simulink model "MPPT_RotEnc_Model1"  (R2018b)
settings: Solver=VariableStepAuto  StartTime=0.0  StopTime=1  RelTol=1e-3  AbsTol=1e-3  EnableMultiTasking=on
values from neighbouring files (symbols this model uses):
  ADC = 1024/5    (= 204.8)    [MPPT_RotEnc_Model.m]
  Cb = 400e-6    (= 0.0004)    [MPPT_RotEnc_Model.m]
  f = 10000    [MPPT_RotEnc_Model.m]
  lambda_pm = 1    [MPPT_RotEnc_Model.m]
  Lb = 1e-3    (= 0.001)    [MPPT_RotEnc_Model.m]
  Ls = 1    [MPPT_RotEnc_Model.m]
  p = 1    [MPPT_RotEnc_Model.m]
  R1 = 200e3    (= 200000)    [MPPT_RotEnc_Model.m]
  R2 = 100e3    (= 100000)    [MPPT_RotEnc_Model.m]
  Rl = 100    [MPPT_RotEnc_Model.m]
  Rs = 1    [MPPT_RotEnc_Model.m]
  Te = 1    [MPPT_RotEnc_Model.m]
  Wc = 1    [MPPT_RotEnc_Model.m]
libraries: powerlib x16, fl_lib x9, nesl_utility x5, elec_lib x1, pe_lib x1
settings Model: Creator=Cyrus  LastModifiedBy=Cyrus
settings SolverCC: AutoScaleAbsTol=off
settings DataIOCC: LimitDataPoints=on  MaxDataPoints=10000
settings OptimizationCC: LifeSpan=inf
settings DebuggingCC: AllowSymbolicDim=off  LibraryContextMissingDiagnostic=none  SFUnexpectedBacktrackingDiag=warning  SFNoUnconditionalDefaultTransitionDiag=warning  SFExecutionAtInitializationDiag=none
settings SFSimCC: SimUseLocalCustomCode=off
settings RTWCC: RTWUseLocalCustomCode=off
settings CodeAppCC: StateflowObjectComments=on
settings GRTTargetCC: TargetLangStandard=C89/C90 (ANSI)  GeneratePreprocessorConditionals=Disable all
settings ConfigComp: CovMetricSettings=dw  CovHtmlReporting=on  CovSaveCumulativeToWorkspaceVar=on  CovSaveSingleToWorkspaceVar=on  CovExternalEMLEnable=off  CovSFcnEnable=off
settings SimscapeCC: SimscapeLogType=all  SimscapeLogDataHistory=10000

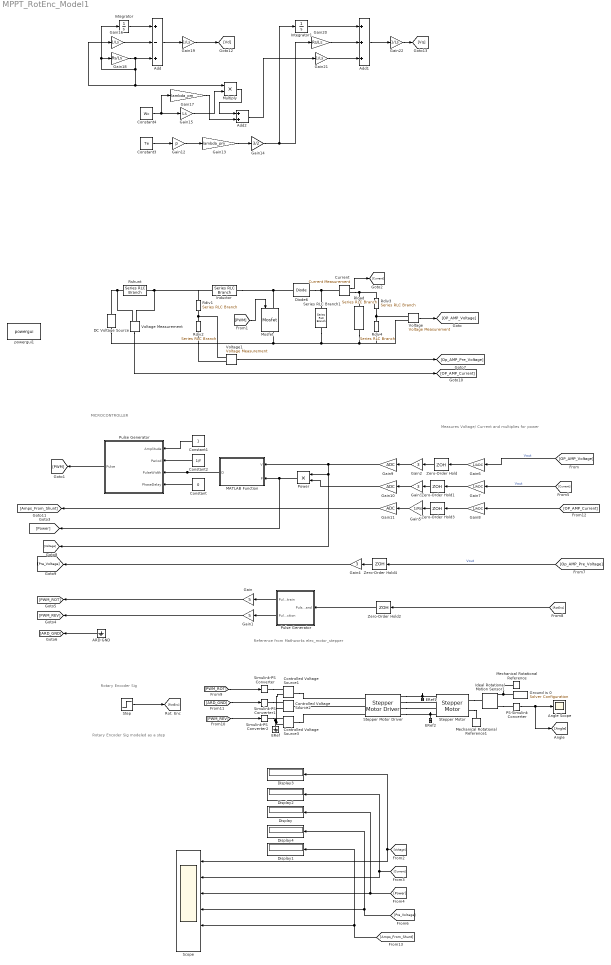
== system MPPT_RotEnc_Model1 ==
  note: Measures Voltage/ Current and multiplies for power
  note: Reference from Mathworks elec_motor_stepper
  note: Rotary Encoder Sig modeled as a step
  note: MICROCONTROLLER
  note: Rotary Encoder Sig
  " Pulse Generator" : Subsystem
  "ARD GND " : Ground
  Add : Sum  Inputs=+-+
  Add1 : Sum  Inputs=+++
  Add2 : Sum
  "Angle Scope " : Scope
  Constant : Constant  Value=0
  Constant1 : Constant
  Constant2 : Constant  Value=1/f
  Constant3 : Constant  Value=Te
  Constant4 : Constant  Value=Wc
  Controlled Voltage Source1 : fl_lib/Electrical/Electrical Sources/Controlled Voltage Source
  Controlled Voltage Source2 : fl_lib/Electrical/Electrical Sources/Controlled Voltage Source
  Controlled Voltage Source3 : fl_lib/Electrical/Electrical Sources/Controlled Voltage Source
  Current : powerlib/Measurements/Current Measurement  PhasorSimulation=off  OutputType=Complex  PSBequivalent=0
  DC Voltage Source : powerlib/Electrical Sources/DC Voltage Source  Amplitude=5  Measurements=None
  Diode6 : powerlib/Power Electronics/Diode  Ron=0.001  Lon=0  Vf=0.8  IC=0  UseSnubber=0  Rs=0  Cs=0  Measurements=off
  Display{,1..4} (5 alike) : Display
  ERef : fl_lib/Electrical/Electrical Elements/Electrical Reference
      settings: SourceProductName=Foundation Library
  ERef1 : fl_lib/Electrical/Electrical Elements/Electrical Reference
      settings: SourceProductName=Foundation Library
  ERef2 : fl_lib/Electrical/Electrical Elements/Electrical Reference
      settings: SourceProductName=Foundation Library
  Gain : Gain  Gain=5
  Gain1 : Gain  Gain=5
  Gain10 : Gain  Gain=ADC
  Gain11 : Gain  Gain=ADC
  Gain12 : Gain  Gain=p
  Gain13 : Gain  Gain=lambda_pm
  Gain14 : Gain  Gain=3/2
  Gain15 : Gain  Gain=Ls
  Gain{16,19,21..22} (4 alike) : Gain  Gain=1/Ls
  Gain17 : Gain  Gain=lambda_pm
  Gain18 : Gain  Gain=Rs/Ls
  Gain2 : Gain  Gain=3
  Gain20 : Gain  Gain=Rs/Ls
  Gain3 : Gain  Gain=3
  Gain4 : Gain  Gain=3
  Gain5 : Gain  Gain=1/Rs
  Gain6 : Gain  Gain=1/ADC
  Gain7 : Gain  Gain=1/ADC
  Gain8 : Gain  Gain=1/ADC
  Gain9 : Gain  Gain=ADC
  "Ground is 0 " : nesl_utility/Solver Configuration  PhysicalDomain=network_engine_domain  SubClassName=solver  LeftPortType=input  RightPortType=generic  Tones=[]  Harmonics=[]  SimulateNoise=off  Profile=off  UseLocalSampling=off  EnableSwitchedLinearOptims=on  FrequencyDomain=off  UseCCode=off  RelTol=0.001  AbsTol=1e-06  MinStep=1e-09  ToWorkspace=off  RevertToSquareIcSolve=off  NumHomotopyIterations=100  PhasorMode=off  PhasorModeNumHarmonics=1  DoDC=off  ResidualTolerance=1e-9  UseLocalSolver=off  LocalSolverChoice=NE_BACKWARD_EULER_ADVANCER  LocalSolverSampleTime=.001  DoFixedCost=off  MaxNonlinIter=3  MaxModeIter=2  LinearAlgebra=auto  EquationFormulation=NE_TIME_EF  DelaysMemoryBudget=1024  AutomaticFiltering=on  FilteringTimeConstant=0.001  PartitionStorageMethod=AS_NEEDED  PartitionMemoryBudget=1024
  Ideal Rotational Motion Sensor1 : fl_lib/Mechanical/Mechanical Sensors/Ideal Rotational Motion Sensor  offset=0 rad
  "Inductor " : powerlib/Elements/Series RLC Branch  LConnTagsString=__new0  RConnTagsString=__new0  BranchType=L  Resistance=1  Inductance=Lb  SetiL0=off  InitialCurrent=0  Capacitance=1e-6  Setx0=off  InitialVoltage=0  Measurements=None
  Integrator : Integrator
  Integrator1 : Integrator
  MATLAB Function : MATLAB Function  TreatAsAtomicUnit=on
  Mechanical Rotational Reference : fl_lib/Mechanical/Rotational Elements/Mechanical Rotational Reference
  Mechanical Rotational Reference1 : fl_lib/Mechanical/Rotational Elements/Mechanical Rotational Reference
  Mosfet : powerlib/Power Electronics/Mosfet  Ron=0.1  Lon=0  Rd=0.01  Vfd=0  IC=0  Rs=1e5  Cs=inf  Measurements=on
  Multiply : Product
  PS-Simulink Converter : nesl_utility/PS-Simulink Converter  PhysicalDomain=network_engine_domain  SubClassName=ps_output  LeftPortType=input  RightPortType=output  PseudoPeriodic=off  Frequencies=[]  Unit=1  AffineConversion=off
  "Power " : Product
  Pulse Generator : Subsystem  mask{f=20}
      mask prompts: f "Pulse rate"
  Rdiv1 : powerlib/Elements/Series RLC Branch  LConnTagsString=__new0  RConnTagsString=__new0  BranchType=R  Resistance=R1  Inductance=1e-3  SetiL0=off  InitialCurrent=0  Capacitance=1e-6  Setx0=off  InitialVoltage=0  Measurements=None
  Rdiv2 : powerlib/Elements/Series RLC Branch  LConnTagsString=__new0  RConnTagsString=__new0  BranchType=R  Resistance=R2  Inductance=1e-3  SetiL0=off  InitialCurrent=0  Capacitance=1e-6  Setx0=off  InitialVoltage=0  Measurements=None
  Rdiv3 : powerlib/Elements/Series RLC Branch  LConnTagsString=__new0  RConnTagsString=__new0  BranchType=R  Resistance=R1  Inductance=1e-3  SetiL0=off  InitialCurrent=0  Capacitance=1e-6  Setx0=off  InitialVoltage=0  Measurements=None
  Rdiv4 : powerlib/Elements/Series RLC Branch  LConnTagsString=__new0  RConnTagsString=__new0  BranchType=R  Resistance=R2  Inductance=1e-3  SetiL0=off  InitialCurrent=0  Capacitance=1e-6  Setx0=off  InitialVoltage=0  Measurements=None
  Rload : powerlib/Elements/Series RLC Branch  LConnTagsString=__new0  RConnTagsString=__new0  BranchType=R  Resistance=Rl  Inductance=1e-3  SetiL0=off  InitialCurrent=0  Capacitance=1e-6  Setx0=off  InitialVoltage=0  Measurements=None
  Rshunt : powerlib/Elements/Series RLC Branch  LConnTagsString=__new0  RConnTagsString=__new0  BranchType=R  Resistance=Rs  Inductance=1e-3  SetiL0=off  InitialCurrent=0  Capacitance=1e-6  Setx0=off  InitialVoltage=0  Measurements=None
  Scope : Scope  NumInputPorts=6
  Series RLC Branch1 : powerlib/Elements/Series RLC Branch  LConnTagsString=__new0  RConnTagsString=__new0  BranchType=C  Resistance=1  Inductance=1e-3  SetiL0=off  InitialCurrent=0  Capacitance=Cb  Setx0=off  InitialVoltage=0  Measurements=None
  Simulink-PS Converter : nesl_utility/Simulink-PS Converter  PhysicalDomain=network_engine_domain  SubClassName=ps_input  LeftPortType=input  RightPortType=output  PseudoPeriodic=off  Frequencies=[]  NoiseDistribution=none  NoiseParameters=[]  Unit=1  AffineConversion=on  FilteringAndDerivatives=provide  SimscapeFilterOrder=1  InputFilterTimeConstant=0.001  UdotUserProvided=0
  Simulink-PS Converter1 : nesl_utility/Simulink-PS Converter  PhysicalDomain=network_engine_domain  SubClassName=ps_input  LeftPortType=input  RightPortType=output  PseudoPeriodic=off  Frequencies=[]  NoiseDistribution=none  NoiseParameters=[]  Unit=1  AffineConversion=on  FilteringAndDerivatives=provide  SimscapeFilterOrder=1  InputFilterTimeConstant=0.001  UdotUserProvided=0
  Simulink-PS Converter2 : nesl_utility/Simulink-PS Converter  PhysicalDomain=network_engine_domain  SubClassName=ps_input  LeftPortType=input  RightPortType=output  PseudoPeriodic=off  Frequencies=[]  NoiseDistribution=none  NoiseParameters=[]  Unit=1  AffineConversion=on  FilteringAndDerivatives=provide  SimscapeFilterOrder=1  InputFilterTimeConstant=0.001  UdotUserProvided=0
  Step : Step  Time=.5  Before=10  After=10  SampleTime=0
  Stepper Motor : elec_lib/Actuators & Drivers/Rotational Actuators/Stepper Motor  step_or_av=1  w_vec=[0, 1000, 3000] rpm  T_vec=[2, 2, 1] N*m  assert_if_slipping=0  J_total=1e-4 kg*m^2  max_step_rate=10 Hz  Ra=0.55 Ohm  La=1.5e-3 H  Km=0.19 N*m/A  Td=0 N*m  Rm=inf Ohm  Step=1.8 deg  J=4.5e-5 kg*m^2  B=8.0e-4 N*m/(rad/s)  speed0=0 rpm  theta0=0 deg  alpha=[.00393, .00393] 1/K  Tmeas=25 degC  T_vec2=[1.7, 1.7, .85] N*m  Tmeas2=125 degC  half_stepping=0  thermal_masses=[100, 100] J/K  initial_temperatures=[25, 25] degC  rotor_thermal_mass=50 J/K  rotor_initial_temperature=25 degC  Rm_percent_rotor=90
      settings: SourceProductName=Simscape Electronics  SourceProductBaseCode=SN
  Stepper Motor Driver : pe_lib/Machines/Stepper Motor and Driver/Stepper Motor Driver  step_or_av=1  step_rate_per_volt=10 Hz/V  Venable=2.5 V  Vreverse=2.5 V  Vm=10 V  half_stepping=0
      settings: SourceProductName=Simscape Power Systems  SourceProductBaseCode=PS
  Voltage : powerlib/Measurements/Voltage Measurement  PhasorSimulation=off  OutputType=Magnitude  PSBequivalent=0
  Voltage Measurement : powerlib/Measurements/Voltage Measurement  PhasorSimulation=off  OutputType=Complex  PSBequivalent=0
  Voltage1 : powerlib/Measurements/Voltage Measurement  PhasorSimulation=off  OutputType=Magnitude  PSBequivalent=0
  Zero-Order Hold{,1..4} (5 alike) : ZeroOrderHold  SampleTime=1e-6
  powergui1 : powerlib/powergui  Priority=1  SimulationMode=Continuous  SampleTime=50e-6  frequency=60  Iterations=50  frequencyindice=0  Pbase=100e6  ErrMax=1e-4  UnitsV=kV  UnitsW=MW  buscounter=0  FunctionMessages=off  echomessages=off  EnableUseOfTLC=off  CurrentSourceSwitches=off  DisableSnubberDevices=off  DisableRonSwitches=off  DisableVfSwitches=off  DisplayEquations=off  SolverType=Tustin/Backward Euler (TBE)  Interpol=off  ExternalGateDelay=off  methode=off  Ts=100  x0status=blocks  SPID=on  SwTol=0  HookPort=off  RestoreLinks=warning  ResistiveCurrentMeasurement=off  Frange=[0:2:500]  Ylog=off  Xlog=on  ShowGrid=off  save=off  variable=ZData  structure=0  ZoomFFT=off  StartTime=0.0  cycles=1  DisplayStyle=1  fundamental=60  FreqAxis=off  MaxFrequency=1000  frequencyindicesteady=1  RmsSteady=1  display=off
  wires:
  [OP_AMP_Voltage] -> Gain6/1  "Vout"
  [Voltage] -> Scope/1, Display3/1
  [Current] -> Display2/1, Scope/2
  [Power] -> Display/1, Scope/3
  [Current] -> Gain7/1  "Vout"
  Voltage/1 -> [OP_AMP_Voltage]
  Current/1 -> [Current]
  Zero-Order Hold1/1 -> Gain3/1
  Zero-Order Hold/1 -> Gain2/1
  "Power "/1 -> MATLAB Function/2(P), [Power]
  Constant/1 -> " Pulse Generator"/4(PhaseDelay)
  Constant1/1 -> " Pulse Generator"/1(Amplitude)
  Constant2/1 -> " Pulse Generator"/2(Period)
  [PWM] -> Mosfet/1
  " Pulse Generator"/1(Pulse) -> [PWM]
  MATLAB Function/1(D) -> " Pulse Generator"/3(PulseWidth)
  [ARD_GND] -> Simulink-PS Converter1/1
  [PWM_ROT] -> Simulink-PS Converter/1
  [PWM_REV] -> Simulink-PS Converter2/1
  PS-Simulink Converter/1 -> [Angle], "Angle Scope "/1
  [RotEnc] -> Zero-Order Hold2/1
  "ARD GND "/1 -> [ARD_GND]
  Pulse Generator/1(Pulse train) -> Gain/1
  Pulse Generator/2(Pulse direction) -> Gain1/1
  Gain/1 -> [PWM_ROT]
  Gain1/1 -> [PWM_REV]
  Zero-Order Hold2/1 -> Pulse Generator/1(Pulse  demand)
  Step/1 -> [RotEnc]
  Voltage1/1 -> [Op_AMP_Pre_Voltage]
  [Pre_Voltage] -> Display4/1, Scope/4
  Gain4/1 -> [Pre_Voltage]
  [Op_AMP_Pre_Voltage] -> Zero-Order Hold4/1  "Vout"
  Voltage Measurement/1 -> [OP_AMP_Current]
  [OP_AMP_Current] -> Gain8/1
  Zero-Order Hold3/1 -> Gain5/1
  [Amps_From_Shunt] -> Display1/1, Scope/5
  Zero-Order Hold4/1 -> Gain4/1
  Gain2/1 -> Gain9/1
  Gain3/1 -> Gain10/1
  Gain5/1 -> Gain11/1
  Gain9/1 -> "Power "/1, [Voltage], MATLAB Function/1(V)
  Gain10/1 -> "Power "/2
  Gain11/1 -> [Amps_From_Shunt]
  Constant3/1 -> Gain12/1
  Gain12/1 -> Gain13/1
  Gain13/1 -> Gain14/1
  Constant4/1 -> Gain15/1, Gain17/1
  Integrator/1 -> Add/1
  Gain16/1 -> Add/2
  Add/1 -> Gain19/1
  Gain19/1 -> [Vd]
  Gain18/1 -> Gain16/1, Multiply/1, Gain18/1, Integrator/1, Add/3
  Gain14/1 -> Gain20/1, Integrator1/1
  Integrator1/1 -> Add1/1
  Gain20/1 -> Add1/2
  Gain21/1 -> Add1/3
  Gain15/1 -> Multiply/2
  Add1/1 -> Gain22/1
  Gain22/1 -> [Vq]
  Multiply/1 -> Add2/1
  Gain17/1 -> Add2/2
  Add2/1 -> Gain21/1
  Gain6/1 -> Zero-Order Hold/1
  Gain7/1 -> Zero-Order Hold1/1
  Gain8/1 -> Zero-Order Hold3/1
  connections:
  Diode6/RConn1 -- Current/LConn1 -- Series RLC Branch1/LConn1
  "Inductor "/RConn1 -- Mosfet/LConn1 -- Diode6/LConn1
  Rshunt/RConn1 -- Voltage Measurement/LConn2 -- Rdiv1/LConn1 -- "Inductor "/LConn1
  Series RLC Branch1/RConn1 -- Voltage/LConn2 -- Rdiv4/RConn1 -- Rload/RConn1 -- Voltage1/LConn2 -- Rdiv2/RConn1 -- DC Voltage Source/LConn1 -- Mosfet/RConn1
  DC Voltage Source/RConn1 -- Voltage Measurement/LConn1 -- Rshunt/LConn1
  ERef/LConn1 -- Controlled Voltage Source2/RConn2 -- Controlled Voltage Source1/RConn2 -- Controlled Voltage Source3/RConn2
  Mechanical Rotational Reference/LConn1 -- "Ground is 0 "/RConn1 -- Ideal Rotational Motion Sensor1/RConn1
  Simulink-PS Converter1/RConn1 -- Controlled Voltage Source2/RConn1
  Stepper Motor Driver/RConn4 -- ERef2/LConn1 -- Stepper Motor/LConn4
  Simulink-PS Converter/RConn1 -- Controlled Voltage Source1/RConn1
  Stepper Motor/RConn1 -- Ideal Rotational Motion Sensor1/LConn1
  Controlled Voltage Source1/LConn1 -- Stepper Motor Driver/LConn1
  Stepper Motor Driver/RConn3 -- Stepper Motor/LConn3
  Stepper Motor/RConn2 -- Mechanical Rotational Reference1/LConn1
  Stepper Motor Driver/RConn2 -- Stepper Motor/LConn2
  Stepper Motor Driver/RConn1 -- ERef1/LConn1 -- Stepper Motor/LConn1
  Simulink-PS Converter2/RConn1 -- Controlled Voltage Source3/RConn1
  Controlled Voltage Source2/LConn1 -- Stepper Motor Driver/LConn2
  Ideal Rotational Motion Sensor1/RConn3 -- PS-Simulink Converter/LConn1
  Controlled Voltage Source3/LConn1 -- Stepper Motor Driver/LConn3
  Rdiv1/RConn1 -- Voltage1/LConn1 -- Rdiv2/LConn1
  Current/RConn1 -- Rdiv3/LConn1 -- Rload/LConn1
  Rdiv3/RConn1 -- Voltage/LConn1 -- Rdiv4/LConn1

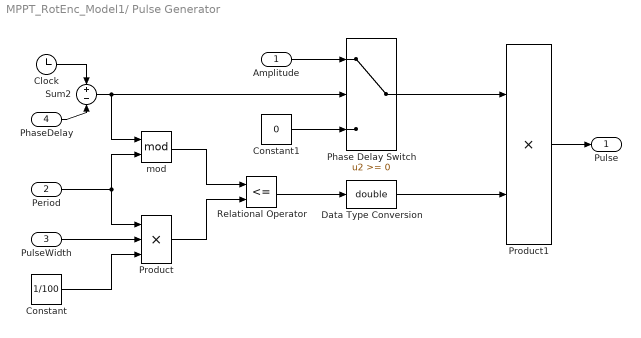
== system MPPT_RotEnc_Model1/ Pulse Generator ==
  Amplitude : Inport
  Period : Inport  Port=2
  PulseWidth : Inport  Port=3
  PhaseDelay : Inport  Port=4
  Clock : Clock
  Constant : Constant  Value=1/100
  Constant1 : Constant  Value=0
  Data Type Conversion : DataTypeConversion  OutDataTypeStr=double
  Phase Delay Switch : Switch
  Product : Product  Inputs=3  RndMeth=Zero
  Product1 : Product  RndMeth=Zero
  Relational Operator : RelationalOperator  Operator=<=  RndMeth=Nearest
  Sum2 : Sum  Inputs=+-
  mod : Math  Operator=mod  SaturateOnIntegerOverflow=on
  Pulse : Outport
  wires:
  Product/1 -> Relational Operator/2
  Product1/1 -> Pulse/1
  Data Type Conversion/1 -> Product1/2
  Relational Operator/1 -> Data Type Conversion/1
  Constant/1 -> Product/3
  PulseWidth/1 -> Product/2
  mod/1 -> Relational Operator/1
  Period/1 -> Product/1, mod/2
  Clock/1 -> Sum2/1
  PhaseDelay/1 -> Sum2/2
  Sum2/1 -> mod/1, Phase Delay Switch/2
  Amplitude/1 -> Phase Delay Switch/1
  Constant1/1 -> Phase Delay Switch/3
  Phase Delay Switch/1 -> Product1/1

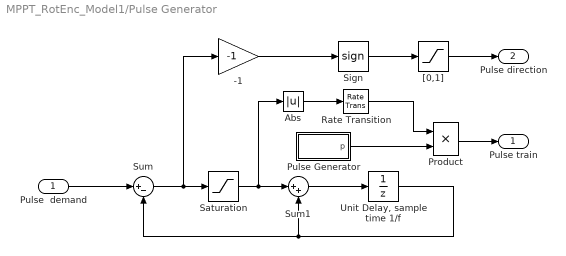
== system MPPT_RotEnc_Model1/Pulse Generator ==
  Pulse  demand : Inport  SampleTime=1/f
  -1 : Gain  Gain=-1
  Abs : Abs
  Product : Product  SaturateOnIntegerOverflow=on  InputSameDT=on  OutDataTypeStr=Inherit: Same as first input
  Pulse Generator : Subsystem
  Rate Transition : RateTransition  Deterministic=off
  Saturation : Saturate  UpperLimit=1  LowerLimit=-1
  Sign : Signum
  Sum : Sum  Inputs=|+-
  Sum1 : Sum  Inputs=|++
  "Unit Delay, sample time 1/f" : UnitDelay  SampleTime=1/f
  "[0,1]" : Saturate  UpperLimit=1  LowerLimit=0
  Pulse train : Outport
  Pulse direction : Outport  Port=2
  wires:
  "[0,1]"/1 -> Pulse direction/1
  -1/1 -> Sign/1
  "Unit Delay, sample time 1/f"/1 -> Sum/2, Sum1/2
  Pulse  demand/1 -> Sum/1
  Sum/1 -> -1/1, Saturation/1
  Saturation/1 -> Sum1/1, Abs/1
  Sum1/1 -> "Unit Delay, sample time 1/f"/1
  Sign/1 -> "[0,1]"/1
  Product/1 -> Pulse train/1
  Abs/1 -> Rate Transition/1
  Pulse Generator/1(p) -> Product/2
  Rate Transition/1 -> Product/1

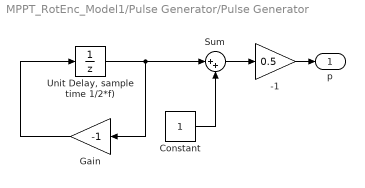
== system MPPT_RotEnc_Model1/Pulse Generator/Pulse Generator ==
  -1 : Gain  Gain=0.5
  Constant : Constant  SampleTime=1/(2*f)
  Gain : Gain  Gain=-1
  Sum : Sum  Inputs=|++
  "Unit Delay, sample time 1/2*f)" : UnitDelay  InitialCondition=-1  SampleTime=1/(2*f)
  p : Outport
  wires:
  "Unit Delay, sample time 1/2*f)"/1 -> Gain/1, Sum/1
  Gain/1 -> "Unit Delay, sample time 1/2*f)"/1
  Constant/1 -> Sum/2
  Sum/1 -> -1/1
  -1/1 -> p/1

== matlab function MPPT_RotEnc_Model1/MATLAB Function ==
  data: V input; P input; D output
function D = MPPT_TRACKING(V,P)
%%================================
%% PERTURB AND OBSERVE ALGORITHM MMPT
%%================================
%% LOCAL VARIABLES USED FOR STORING OLD VALUES

    dD = .0001 ;                  %DUTY CYCLE INCREMENT/DECREMENT
    persistent old_D             %MEMORY, OLD DUTY CYCLE 
    persistent old_P         %MEMORY, OLD POWER 
    persistent old_V         %MEMORY, OLD VOLTAGE

    if isempty (old_D)
        old_D = 30;              %INITIAL DUTY CYCLE IS 20%
        old_P = 1;
        old_V = 5;
    end

    if (V >= 15)
        D = old_D - dD;
    elseif (V <= 10) 
        D = old_D + dD;    
    elseif (V > old_V)
        if (P > old_P)
           D = old_D + dD; 
        else
           D = old_D - dD; 
        end
    elseif (V < old_V)
         if (P > old_P)
           D = old_D - dD; 
        else
           D = old_D + dD; 
         end
    else
         D = old_D;
    end
    
    old_P = P;
    old_D = D;
    old_V = V;
